simulink model "Modulation_Example_GMSK_Simulink"  (R2020b)
settings: Solver=VariableStepAuto  StartTime=0.0  StopTime=352  RelTol=1e-3
libraries: commanapbnd3 x2
settings Model: Creator=user  LastModifiedBy=giusp

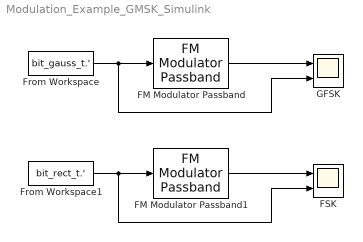
== system Modulation_Example_GMSK_Simulink ==
  FM Modulator Passband : commanapbnd3/FM Modulator Passband  Fc=1/4  Ph=0  Kc=1/8
      settings: SourceProductBaseCode=CM
  FM Modulator Passband1 : commanapbnd3/FM Modulator Passband  Fc=1/4  Ph=0  Kc=1/8
      settings: SourceProductBaseCode=CM
  FSK : Scope  NumInputPorts=2
  From Workspace : FromWorkspace  VariableName=bit_gauss_t.'  SampleTime=0.001
  From Workspace1 : FromWorkspace  VariableName=bit_rect_t.'  SampleTime=0.001
  GFSK : Scope  NumInputPorts=2
  wires:
  From Workspace/1 -> GFSK/2, FM Modulator Passband/1
  FM Modulator Passband/1 -> GFSK/1
  From Workspace1/1 -> FSK/2, FM Modulator Passband1/1
  FM Modulator Passband1/1 -> FSK/1
